simulink model "43_BusNetworkElectricityTransmissionModel"  (R2023b)
settings: Solver=VariableStepAuto  StartTime=0.0  StopTime=0.8  RelTol=1e-3
model workspace (MAT data in the model file):
  BESS_Fp_KDroop = 0.025
  BESS_KSI = 817
  BESS_PWM_fs = 560
  BESS_P_Ki = 0.5
  BESS_P_Kp = 0.0636
  BESS_Pnom = 3000000
  BESS_Q_Ki = 1
  BESS_Q_Kp = 0.0257
  BESS_Vd_Ki = 850
  BESS_Vd_Kp = 0.216
  BESS_Vnom = 1000
  BESS_Vq_KDroop = 0.025
  BESS_Vq_Ki = 850
  BESS_Vq_Kp = 0.216
  Compensation_Ki = 30
  Compensation_Kp = 3
  DC_Ki = 400
  DC_Kp = 8
  F = 0.01
  Flux_min = 0.5
  Grid_Freq_PWM = 2700
  Grid_Ireg_Ki = 5
  Grid_Ireg_Kp = 0.83
  Grid_Ireg_lim = 1.1
  Grid_Modindex_Upper = 1.1
  Grid_conv_Imax = 0.8
  H = 0.685
  Idref_max = 0.9
  Iqref_Tc = 0.3
  Ki_Var = 0.05
  Ki_Vreg = 20
  Ksh = 1.1
  L_pu = 0.3
  Llr = 0.16
  Lls = 0.18
  Lm = 2.9
  LowLoad_P = 130
  Nb_wt = 6
  P_mech = 1080000
  PeakShav_P = 200
  Pitch_Ki = 0
  Pitch_Kp = 150
  Pitch_Max = 27
  Pitch_Tc = 0.01
  Pitch_rate = 10
  Q_Filt = 50
  R_pu = 0.003
  Rotor_Freq_PWM = 1620
  Rotor_Ireg_Ki = 8
  Rotor_Ireg_Kp = 0.6
  Rotor_Ireg_lim = 0.1
  Rotor_Modindex_Upper = 2
  Rr = 0.016
  Rs = 0.023
  SOCBESS : Simulink.Parameter (value not decoded)
  T_set = 0.0001
  Tp = 5e-05
  Ts = 5e-06
  Var_C_Filt = 720000
  Var_reg_max = 1.1
  Var_reg_min = 0.9
  WT_Coeff = [0.645 116 0.4 5 21 0.00912 0.08 0.035]
  WT_H = 4.32
  WT_IGBTRon = 5.931
  WT_Param = [91.204 10143]
  Wind_Freq_Filt = 10000
  Wind_Freq_nom = 60
  Wind_P_nom = 1200000
  Wind_Rotor_V_nom = 1950
  Wind_V_nom = 500
  Zeta_Filt = 0.707106781187
  init = [-0.2 0 0 0 0 0 0 0]
  p = 3
  torque0 = 0.83
  v_Ki = 0.1
  v_Kp = 3.6
  v_Max = 1.2
  v_Min = 0.7
  v_T = 5
  vreg_max = 1
  wind_VDC_nom = 1150
  wt0 = 1.2
undefined symbols (not defined in the file): D1, D11, Delta, DiscIntNeverNeededParam, Iabc, Ion, Lithium, P, Q, Vabc
libraries: powerlib_extras x156, spsSeriesRLCBranchLib x66, spsLoadFlowBusLib x43, spsThreePhaseSeriesRLCLoadLib x33, spsThreePhaseTransformerTwoWindingsLib x32, spsThreePhaseVIMeasurementLib x30, simulink_extras x30, spsDistributedParametersLineLib x22, spsGenericPowerSystemStabilizerLib x20, spsSynchronousMachinepuStandardLib x10, spsExcitationSystemLib x10, spsHydraulicTurbineandGovernorLib x10
(part 7 of 19)

== system 43_BusNetworkElectricityTransmissionModel/South Network/Regulators 2 ==
  m : Inport
  Bus Selector : BusSelector  OutputSignals="dq0 components.Stator voltage  vq (pu),dq0 components.Stator voltage  vd (pu),Mechanical.Rotor speed  wm  (pu),Output active power   Peo (pu)"
  Constant : Constant  Value=0.8
  Constant1 : Constant
  Math Function : Math  Operator=hypot
  Turbine and Excitation Regulators : Subsystem
  Pm : Outport
  Vf : Outport  Port=2
  tag scope: Vm2=global, w2=global
  wires:
  Constant1/1 -> Turbine and Excitation Regulators/4(Vref)
  Turbine and Excitation Regulators/1(Pm) -> Pm/1
  m/1 -> Bus Selector/1
  Turbine and Excitation Regulators/2(Vf) -> Vf/1
  Bus Selector/1 -> Math Function/1  "<Stator voltage  vq (pu)>"
  Math Function/1 -> [Vm2], Turbine and Excitation Regulators/5(Vm)
  Bus Selector/2 -> Math Function/2  "<Stator voltage  vd (pu)>"
  Constant/1 -> Turbine and Excitation Regulators/1(pref)
  Bus Selector/3 -> [w2], Turbine and Excitation Regulators/2(w)  "<Rotor speed  wm  (pu)>"
  Bus Selector/4 -> Turbine and Excitation Regulators/3(Pe 0)  "<Output active power   Peo (pu)>"

== system 43_BusNetworkElectricityTransmissionModel/South Network/Regulators 3 ==
  m : Inport
  Bus Selector : BusSelector  OutputSignals="dq0 components.Stator voltage  vq (pu),dq0 components.Stator voltage  vd (pu),Mechanical.Rotor speed  wm  (pu),Output active power   Peo (pu)"
  Constant : Constant  Value=0.874
  Constant1 : Constant
  Math Function : Math  Operator=hypot
  Turbine and Excitation Regulators : Subsystem
  Pm : Outport
  Vf : Outport  Port=2
  tag scope: Vm3=global, w3=global
  wires:
  Bus Selector/4 -> Turbine and Excitation Regulators/3(Pe 0)  "<Output active power   Peo (pu)>"
  Constant1/1 -> Turbine and Excitation Regulators/4(Vref)
  Bus Selector/3 -> [w3], Turbine and Excitation Regulators/2(w)  "<Rotor speed  wm  (pu)>"
  Turbine and Excitation Regulators/1(Pm) -> Pm/1
  m/1 -> Bus Selector/1
  Turbine and Excitation Regulators/2(Vf) -> Vf/1
  Bus Selector/1 -> Math Function/1  "<Stator voltage  vq (pu)>"
  Math Function/1 -> [Vm3], Turbine and Excitation Regulators/5(Vm)
  Bus Selector/2 -> Math Function/2  "<Stator voltage  vd (pu)>"
  Constant/1 -> Turbine and Excitation Regulators/1(pref)

== system 43_BusNetworkElectricityTransmissionModel/South Network/Regulators 4 ==
  m : Inport
  Bus Selector : BusSelector  OutputSignals="dq0 components.Stator voltage  vq (pu),dq0 components.Stator voltage  vd (pu),Mechanical.Rotor speed  wm  (pu),Output active power   Peo (pu)"
  Constant : Constant  Value=0.842
  Constant1 : Constant
  Math Function : Math  Operator=hypot
  Turbine and Excitation Regulators : Subsystem
  Pm : Outport
  Vf : Outport  Port=2
  tag scope: Vm4=global, w4=global
  wires:
  Bus Selector/4 -> Turbine and Excitation Regulators/3(Pe 0)  "<Output active power   Peo (pu)>"
  Constant1/1 -> Turbine and Excitation Regulators/4(Vref)
  Bus Selector/3 -> [w4], Turbine and Excitation Regulators/2(w)  "<Rotor speed  wm  (pu)>"
  Turbine and Excitation Regulators/1(Pm) -> Pm/1
  m/1 -> Bus Selector/1
  Turbine and Excitation Regulators/2(Vf) -> Vf/1
  Bus Selector/1 -> Math Function/1  "<Stator voltage  vq (pu)>"
  Math Function/1 -> [Vm4], Turbine and Excitation Regulators/5(Vm)
  Bus Selector/2 -> Math Function/2  "<Stator voltage  vd (pu)>"
  Constant/1 -> Turbine and Excitation Regulators/1(pref)

== system 43_BusNetworkElectricityTransmissionModel/South Network/Regulators 5 ==
  m : Inport
  Bus Selector : BusSelector  OutputSignals="dq0 components.Stator voltage  vq (pu),dq0 components.Stator voltage  vd (pu),Mechanical.Rotor speed  wm  (pu),Output active power   Peo (pu)"
  Constant : Constant  Value=0.881
  Constant1 : Constant
  Math Function : Math  Operator=hypot
  Turbine and Excitation Regulators : Subsystem
  Pm : Outport
  Vf : Outport  Port=2
  tag scope: Vm5=global, w5=global
  wires:
  Constant1/1 -> Turbine and Excitation Regulators/4(Vref)
  Turbine and Excitation Regulators/1(Pm) -> Pm/1
  m/1 -> Bus Selector/1
  Turbine and Excitation Regulators/2(Vf) -> Vf/1
  Math Function/1 -> [Vm5], Turbine and Excitation Regulators/5(Vm)
  Constant/1 -> Turbine and Excitation Regulators/1(pref)
  Bus Selector/1 -> Math Function/1  "<Stator voltage  vq (pu)>"
  Bus Selector/2 -> Math Function/2  "<Stator voltage  vd (pu)>"
  Bus Selector/4 -> Turbine and Excitation Regulators/3(Pe 0)  "<Output active power   Peo (pu)>"
  Bus Selector/3 -> Turbine and Excitation Regulators/2(w), [w5]  "<Rotor speed  wm  (pu)>"

== system 43_BusNetworkElectricityTransmissionModel/South Network/Regulators 6 ==
  m : Inport
  Bus Selector : BusSelector  OutputSignals="dq0 components.Stator voltage  vq (pu),dq0 components.Stator voltage  vd (pu),Mechanical.Rotor speed  wm  (pu),Output active power   Peo (pu)"
  Constant : Constant  Value=0.847
  Constant1 : Constant
  Math Function : Math  Operator=hypot
  Turbine and Excitation Regulators : Subsystem
  Pm : Outport
  Vf : Outport  Port=2
  tag scope: Vm6=global, w6=global
  wires:
  Constant1/1 -> Turbine and Excitation Regulators/4(Vref)
  Turbine and Excitation Regulators/1(Pm) -> Pm/1
  m/1 -> Bus Selector/1
  Turbine and Excitation Regulators/2(Vf) -> Vf/1
  Math Function/1 -> [Vm6], Turbine and Excitation Regulators/5(Vm)
  Constant/1 -> Turbine and Excitation Regulators/1(pref)
  Bus Selector/1 -> Math Function/1  "<Stator voltage  vq (pu)>"
  Bus Selector/2 -> Math Function/2  "<Stator voltage  vd (pu)>"
  Bus Selector/4 -> Turbine and Excitation Regulators/3(Pe 0)  "<Output active power   Peo (pu)>"
  Bus Selector/3 -> Turbine and Excitation Regulators/2(w), [w6]  "<Rotor speed  wm  (pu)>"

== system 43_BusNetworkElectricityTransmissionModel/ 41.4 MW Wind Generation/41.4 MW Wind Farm/10.35 MW Wind Turbine 1 ==
  " base " : Gain  Gain=-P_mech/Wind_P_nom  SaturateOnIntegerOverflow=on  OutDataTypeStr=Inherit: Same as input  ParamDataTypeStr=Inherit: Same as input
  Asynchronous Machine pu Units : spsAsynchronousMachinepuUnitsLib/Asynchronous Machine pu Units  RotorType=Wound  PresetModel=No  MechanicalLoad=Torque Tm  ShowDetailedParameters=on  ReferenceFrame=Rotor  Units=pu  MeasurementBus=off  NominalParameters=[1.15e7 500 60]  VoltageRatio=1  Stator=[0.023 0.18]  Rotor=[0.016 0.16]  Cage1=[0.01909 0.0397]  Cage2=[0.01909 0.0397]  Lm=2.9  Mechanical=[0.685,0.01,3]  PolePairs=2  InitialConditions="[ -0.2,0   0,0,0   0,0,0 ]"  SimulateSaturation=off  Saturation="[0.212,0.4201,0.8125,1.0979,1.4799,2.2457,3.2586,4.5763,6.4763 ;   0.5,0.7,0.9,1,1.1,1.2 ,1.3,1.4,1.5]"  LoadFlowParameters=0  TsPowergui=0  TsBlock=-1  IterativeModel=Trapezoidal non iterative  IterativeDiscreteModel=Trapezoidal non iterative  Pmec=1.08e6
      settings: LibrarySourceBlock=|
      | sps_lib/Electrical Machines/Asynchronous Machine
      | pu Units
  Bus Selector : BusSelector  OutputSignals=Stator measurements.Stator current is_a (pu),Stator measurements.Stator current is_b (pu),Stator measurements.Stator current is_c (pu),Rotor measurements.Rotor current ir_a (pu),Rotor measurements.Rotor current ir_b (pu),Rotor measurements.Rotor current ir_c (pu),Mechanical.Electromagnetic torque Te (pu),Mechanical.Rotor speed (wm),Mechanical.Rotor angle thetam (rad)
  Mux : Mux  Inputs=3
  Mux1 : Mux  Inputs=3
  Series RLC Branch4 : spsSeriesRLCBranchLib/Series RLC Branch  LConnTagsString=__new0  RConnTagsString=__new0  BranchType=C  Resistance=1  Inductance=1e-3  SetiL0=off  InitialCurrent=0  Capacitance=4e-3  Setx0=on  InitialVoltage=1175  Measurements=None
  Three-Phase Series RLC Branch : spsThreePhaseSeriesRLCBranchLib/Three-Phase Series RLC Branch  LConnTagsString=A|B|C  RConnTagsString=A|B|C  BranchType=RL  Resistance=(Wind_V_nom^2/Wind_P_nom)*R_pu  Inductance=(Wind_V_nom^2/Wind_P_nom/(2*pi*Wind_Freq_nom))*L_pu  Capacitance=1e-6  Measurements=None
  Three-Phase Transformer (Two Windings) : spsThreePhaseTransformerTwoWindingsLib/Three-Phase Transformer (Two Windings)  Winding1Connection=Y  Winding2Connection=Y  CoreType=Three single-phase transformers  SetSaturation=off  Hysteresis=off  DataFile='hysteresis'  SetInitialFlux=off  Measurements=None  UNITS=pu  NominalPower=[1.15e7, 60 ]  Winding1="[ 500, 0,0  ]"  Winding2=[ 1950 , 0 , 0 ]  Rm=500  Lm=inf  L0=0.5  Saturation=[ 0,0 ; 0.0024,1.2 ; 1.0,1.52 ]  InitialFluxes=[ 0.8 , -0.8 , 0.7 ]  BreakLoop=off  DiscreteSolver=Trapezoidal iterative  DataType=off  TransfoNumber=1
  Three-Phase V-I Measurement5 : spsThreePhaseVIMeasurementLib/Three-Phase V-I Measurement  VoltageMeasurement=phase-to-ground  SetLabelV=on  LabelV=Rotor_Vabc_WT1  Vpu=on  VpuLL=off  CurrentMeasurement=no  SetLabelI=on  LabelI=Iabc_WT1  Ipu=on  Pbase=2*1.8/0.9  Vbase=Wind_Rotor_V_nom  OutputType=Complex  PhasorSimulation=off  PSBequivalent=0
  Three-Phase V-I Measurement6 : spsThreePhaseVIMeasurementLib/Three-Phase V-I Measurement  VoltageMeasurement=phase-to-ground  SetLabelV=on  LabelV=Grid_conv_Vabc_WT1  Vpu=on  VpuLL=off  CurrentMeasurement=yes  SetLabelI=on  LabelI=Grid_conv_Iabc_WT1  Ipu=on  Pbase=1.15e7  Vbase=Wind_V_nom  OutputType=Complex  PhasorSimulation=off  PSBequivalent=0
  Universal Bridge : spsUniversalBridgeLib/Universal Bridge  Arms=3  SnubberResistance=1e3  SnubberCapacitance=inf  Device=IGBT / Diodes  Ron=1e-4/WT_IGBTRon  Lon=0  ForwardVoltages="[  0  0  ]"  ForwardVoltage=0  GTOparameters=[ 10e-6 , 20e-6 ]  IGBTparameters=[ 1e-6 , 2e-6 ]  Measurements=None  Measurements_2=None  converterType=Rectifier
  Universal Bridge1 : spsUniversalBridgeLib/Universal Bridge  Arms=3  SnubberResistance=1e3  SnubberCapacitance=inf  Device=IGBT / Diodes  Ron=1e-4/WT_IGBTRon  Lon=0  ForwardVoltages="[  0  0  ]"  ForwardVoltage=0  GTOparameters=[ 10e-6 , 20e-6 ]  IGBTparameters=[ 1e-6 , 2e-6 ]  Measurements=None  Measurements_2=None  converterType=Rectifier
  Wind Turbine & Generator 1 : Subsystem
  A : PMIOPort  Side=Left
  B : PMIOPort  Port=2  Side=Left
  C : PMIOPort  Port=3  Side=Left
  tag scope: Rotor_Angle_WT1=global, Rotor_Iabc_WT1=global, Rotor_Tem_WT1=global, Rotor_wm_WT1=global, Stator_Iabc_WT1=global, Tshaft_WT1=global, m_WT1=global
  wires:
  [Tshaft_WT1] -> Asynchronous Machine pu Units/1
  Wind Turbine & Generator 1/1(T_shaft (pu)) -> " base "/1
  " base "/1 -> [Tshaft_WT1]
  Asynchronous Machine pu Units/1 -> [m_WT1]
  [Grid_conv_pulses_WT1] -> Universal Bridge1/1
  [Rotor_conv_pulses_WT1] -> Universal Bridge/1
  [Rotor_wm_WT1] -> Wind Turbine & Generator 1/1(Generator speed (pu))
  [m_WT1] -> Bus Selector/1
  Bus Selector/1 -> Mux1/1  "<Stator current is_a (pu)>"
  Bus Selector/2 -> Mux1/2  "<Stator current is_b (pu)>"
  Bus Selector/3 -> Mux1/3  "<Stator current is_c (pu)>"
  Bus Selector/4 -> Mux/1  "<Rotor current ir_a (pu)>"
  Bus Selector/5 -> Mux/2  "<Rotor current ir_b (pu)>"
  Bus Selector/6 -> Mux/3  "<Rotor current ir_c (pu)>"
  Bus Selector/7 -> [Rotor_Tem_WT1]  "<Electromagnetic torque Te (pu)>"
  Bus Selector/8 -> [Rotor_wm_WT1]  "<Rotor speed (wm)>"
  Bus Selector/9 -> [Rotor_Angle_WT1]  "<Rotor angle thetam (rad)>"
  Mux/1 -> [Rotor_Iabc_WT1]
  Mux1/1 -> [Stator_Iabc_WT1]
  connections:
  Asynchronous Machine pu Units/LConn3 -- C/RConn1 -- Three-Phase Series RLC Branch/LConn3
  Three-Phase Series RLC Branch/LConn1 -- A/RConn1 -- Asynchronous Machine pu Units/LConn1
  Three-Phase Transformer (Two Windings)/LConn1 -- Asynchronous Machine pu Units/RConn1
  Three-Phase Transformer (Two Windings)/RConn1 -- Three-Phase V-I Measurement5/LConn1
  Three-Phase Series RLC Branch/LConn2 -- B/RConn1 -- Asynchronous Machine pu Units/LConn2
  Universal Bridge1/LConn3 -- Three-Phase V-I Measurement6/RConn3
  Three-Phase Transformer (Two Windings)/LConn3 -- Asynchronous Machine pu Units/RConn3
  Three-Phase Transformer (Two Windings)/LConn2 -- Asynchronous Machine pu Units/RConn2
  Universal Bridge1/LConn2 -- Three-Phase V-I Measurement6/RConn2
  Universal Bridge/RConn1 -- Series RLC Branch4/LConn1 -- Universal Bridge1/RConn1
  Universal Bridge1/RConn2 -- Series RLC Branch4/RConn1 -- Universal Bridge/RConn2
  Three-Phase Transformer (Two Windings)/RConn2 -- Three-Phase V-I Measurement5/LConn2
  Three-Phase V-I Measurement5/RConn3 -- Universal Bridge/LConn3
  Three-Phase V-I Measurement5/RConn1 -- Universal Bridge/LConn1
  Three-Phase Transformer (Two Windings)/RConn3 -- Three-Phase V-I Measurement5/LConn3
  Three-Phase V-I Measurement6/LConn1 -- Three-Phase Series RLC Branch/RConn1
  Three-Phase Series RLC Branch/RConn2 -- Three-Phase V-I Measurement6/LConn2
  Universal Bridge1/LConn1 -- Three-Phase V-I Measurement6/RConn1
  Three-Phase Series RLC Branch/RConn3 -- Three-Phase V-I Measurement6/LConn3
  Three-Phase V-I Measurement5/RConn2 -- Universal Bridge/LConn2

== system 43_BusNetworkElectricityTransmissionModel/ 41.4 MW Wind Generation/41.4 MW Wind Farm/10.35 MW Wind Turbine 2 ==
  " base " : Gain  Gain=-P_mech/Wind_P_nom  SaturateOnIntegerOverflow=on  OutDataTypeStr=Inherit: Same as input  ParamDataTypeStr=Inherit: Same as input
  Asynchronous Machine pu Units : spsAsynchronousMachinepuUnitsLib/Asynchronous Machine pu Units  RotorType=Wound  PresetModel=No  MechanicalLoad=Torque Tm  ShowDetailedParameters=on  ReferenceFrame=Rotor  Units=pu  MeasurementBus=off  NominalParameters=[1.15e7 500 60]  VoltageRatio=1  Stator=[0.023 0.18]  Rotor=[0.016 0.16]  Cage1=[0.01909 0.0397]  Cage2=[0.01909 0.0397]  Lm=2.9  Mechanical=[0.685,0.01,3]  PolePairs=2  InitialConditions="[ -0.2,0   0,0,0   0,0,0 ]"  SimulateSaturation=off  Saturation="[0.212,0.4201,0.8125,1.0979,1.4799,2.2457,3.2586,4.5763,6.4763 ;   0.5,0.7,0.9,1,1.1,1.2 ,1.3,1.4,1.5]"  LoadFlowParameters=0  TsPowergui=0  TsBlock=-1  IterativeModel=Trapezoidal non iterative  IterativeDiscreteModel=Trapezoidal non iterative  Pmec=1.08e6
      settings: LibrarySourceBlock=|
      | sps_lib/Electrical Machines/Asynchronous Machine
      | pu Units
  Bus Selector : BusSelector  OutputSignals=Stator measurements.Stator current is_a (pu),Stator measurements.Stator current is_b (pu),Stator measurements.Stator current is_c (pu),Rotor measurements.Rotor current ir_a (pu),Rotor measurements.Rotor current ir_b (pu),Rotor measurements.Rotor current ir_c (pu),Mechanical.Electromagnetic torque Te (pu),Mechanical.Rotor speed (wm),Mechanical.Rotor angle thetam (rad)
  Mux : Mux  Inputs=3
  Mux1 : Mux  Inputs=3
  Series RLC Branch4 : spsSeriesRLCBranchLib/Series RLC Branch  LConnTagsString=__new0  RConnTagsString=__new0  BranchType=C  Resistance=1  Inductance=1e-3  SetiL0=off  InitialCurrent=0  Capacitance=4e-3  Setx0=on  InitialVoltage=1175  Measurements=None
  Three-Phase Series RLC Branch : spsThreePhaseSeriesRLCBranchLib/Three-Phase Series RLC Branch  LConnTagsString=A|B|C  RConnTagsString=A|B|C  BranchType=RL  Resistance=(Wind_V_nom^2/Wind_P_nom)*R_pu  Inductance=(Wind_V_nom^2/Wind_P_nom/(2*pi*Wind_Freq_nom))*L_pu  Capacitance=1e-6  Measurements=None
  Three-Phase Transformer (Two Windings) : spsThreePhaseTransformerTwoWindingsLib/Three-Phase Transformer (Two Windings)  Winding1Connection=Y  Winding2Connection=Y  CoreType=Three single-phase transformers  SetSaturation=off  Hysteresis=off  DataFile='hysteresis'  SetInitialFlux=off  Measurements=None  UNITS=pu  NominalPower=[1.15e7, 60 ]  Winding1="[ 500, 0,0  ]"  Winding2=[ 1950 , 0 , 0 ]  Rm=500  Lm=inf  L0=0.5  Saturation=[ 0,0 ; 0.0024,1.2 ; 1.0,1.52 ]  InitialFluxes=[ 0.8 , -0.8 , 0.7 ]  BreakLoop=off  DiscreteSolver=Trapezoidal iterative  DataType=off  TransfoNumber=1
  Three-Phase V-I Measurement5 : spsThreePhaseVIMeasurementLib/Three-Phase V-I Measurement  VoltageMeasurement=phase-to-ground  SetLabelV=on  LabelV=Rotor_Vabc_WT2  Vpu=on  VpuLL=off  CurrentMeasurement=no  SetLabelI=on  LabelI=Iabc_WT1  Ipu=on  Pbase=2*1.8/0.9  Vbase=Wind_Rotor_V_nom  OutputType=Complex  PhasorSimulation=off  PSBequivalent=0
  Three-Phase V-I Measurement6 : spsThreePhaseVIMeasurementLib/Three-Phase V-I Measurement  VoltageMeasurement=phase-to-ground  SetLabelV=on  LabelV=Grid_conv_Vabc_WT2  Vpu=on  VpuLL=off  CurrentMeasurement=yes  SetLabelI=on  LabelI=Grid_conv_Iabc_WT2  Ipu=on  Pbase=1.15e7  Vbase=Wind_V_nom  OutputType=Complex  PhasorSimulation=off  PSBequivalent=0
  Universal Bridge : spsUniversalBridgeLib/Universal Bridge  Arms=3  SnubberResistance=1e3  SnubberCapacitance=inf  Device=IGBT / Diodes  Ron=1e-4/WT_IGBTRon  Lon=0  ForwardVoltages="[  0  0  ]"  ForwardVoltage=0  GTOparameters=[ 10e-6 , 20e-6 ]  IGBTparameters=[ 1e-6 , 2e-6 ]  Measurements=None  Measurements_2=None  converterType=Rectifier
  Universal Bridge1 : spsUniversalBridgeLib/Universal Bridge  Arms=3  SnubberResistance=1e3  SnubberCapacitance=inf  Device=IGBT / Diodes  Ron=1e-4/WT_IGBTRon  Lon=0  ForwardVoltages="[  0  0  ]"  ForwardVoltage=0  GTOparameters=[ 10e-6 , 20e-6 ]  IGBTparameters=[ 1e-6 , 2e-6 ]  Measurements=None  Measurements_2=None  converterType=Rectifier
  Wind Turbine & Generator 1 : Subsystem
  A : PMIOPort  Side=Left
  B : PMIOPort  Port=2  Side=Left
  C : PMIOPort  Port=3  Side=Left
  tag scope: Rotor_Angle_WT2=global, Rotor_Iabc_WT2=global, Rotor_Tem_WT2=global, Rotor_wm_WT2=global, Stator_Iabc_WT2=global, Tshaft_WT2=global, m_WT2=global
  wires:
  [Tshaft_WT2] -> Asynchronous Machine pu Units/1
  Wind Turbine & Generator 1/1(T_shaft (pu)) -> " base "/1
  " base "/1 -> [Tshaft_WT2]
  Asynchronous Machine pu Units/1 -> [m_WT2]
  [Grid_conv_pulses_WT2] -> Universal Bridge1/1
  [Rotor_conv_pulses_WT2] -> Universal Bridge/1
  [Rotor_wm_WT2] -> Wind Turbine & Generator 1/1(Generator speed (pu))
  [m_WT2] -> Bus Selector/1
  Bus Selector/1 -> Mux1/1  "<Stator current is_a (pu)>"
  Bus Selector/2 -> Mux1/2  "<Stator current is_b (pu)>"
  Bus Selector/3 -> Mux1/3  "<Stator current is_c (pu)>"
  Bus Selector/4 -> Mux/1  "<Rotor current ir_a (pu)>"
  Bus Selector/5 -> Mux/2  "<Rotor current ir_b (pu)>"
  Bus Selector/6 -> Mux/3  "<Rotor current ir_c (pu)>"
  Bus Selector/7 -> [Rotor_Tem_WT2]  "<Electromagnetic torque Te (pu)>"
  Bus Selector/8 -> [Rotor_wm_WT2]  "<Rotor speed (wm)>"
  Bus Selector/9 -> [Rotor_Angle_WT2]  "<Rotor angle thetam (rad)>"
  Mux/1 -> [Rotor_Iabc_WT2]
  Mux1/1 -> [Stator_Iabc_WT2]
  connections:
  Asynchronous Machine pu Units/LConn3 -- C/RConn1 -- Three-Phase Series RLC Branch/LConn3
  Three-Phase Series RLC Branch/LConn1 -- A/RConn1 -- Asynchronous Machine pu Units/LConn1
  Three-Phase Transformer (Two Windings)/LConn1 -- Asynchronous Machine pu Units/RConn1
  Three-Phase Transformer (Two Windings)/RConn1 -- Three-Phase V-I Measurement5/LConn1
  Three-Phase Series RLC Branch/LConn2 -- B/RConn1 -- Asynchronous Machine pu Units/LConn2
  Universal Bridge1/LConn3 -- Three-Phase V-I Measurement6/RConn3
  Three-Phase Transformer (Two Windings)/LConn3 -- Asynchronous Machine pu Units/RConn3
  Three-Phase Transformer (Two Windings)/LConn2 -- Asynchronous Machine pu Units/RConn2
  Universal Bridge1/LConn2 -- Three-Phase V-I Measurement6/RConn2
  Universal Bridge/RConn1 -- Series RLC Branch4/LConn1 -- Universal Bridge1/RConn1
  Universal Bridge1/RConn2 -- Series RLC Branch4/RConn1 -- Universal Bridge/RConn2
  Three-Phase Transformer (Two Windings)/RConn2 -- Three-Phase V-I Measurement5/LConn2
  Three-Phase V-I Measurement5/RConn3 -- Universal Bridge/LConn3
  Three-Phase V-I Measurement5/RConn1 -- Universal Bridge/LConn1
  Three-Phase Transformer (Two Windings)/RConn3 -- Three-Phase V-I Measurement5/LConn3
  Three-Phase V-I Measurement6/LConn1 -- Three-Phase Series RLC Branch/RConn1
  Three-Phase Series RLC Branch/RConn2 -- Three-Phase V-I Measurement6/LConn2
  Universal Bridge1/LConn1 -- Three-Phase V-I Measurement6/RConn1
  Three-Phase Series RLC Branch/RConn3 -- Three-Phase V-I Measurement6/LConn3
  Three-Phase V-I Measurement5/RConn2 -- Universal Bridge/LConn2

== system 43_BusNetworkElectricityTransmissionModel/ 41.4 MW Wind Generation/41.4 MW Wind Farm/10.35 MW Wind Turbine 3 ==
  " base " : Gain  Gain=-P_mech/Wind_P_nom  SaturateOnIntegerOverflow=on  OutDataTypeStr=Inherit: Same as input  ParamDataTypeStr=Inherit: Same as input
  Asynchronous Machine pu Units : spsAsynchronousMachinepuUnitsLib/Asynchronous Machine pu Units  RotorType=Wound  PresetModel=No  MechanicalLoad=Torque Tm  ShowDetailedParameters=on  ReferenceFrame=Rotor  Units=pu  MeasurementBus=off  NominalParameters=[1.15e7 500 60]  VoltageRatio=1  Stator=[0.023 0.18]  Rotor=[0.016 0.16]  Cage1=[0.01909 0.0397]  Cage2=[0.01909 0.0397]  Lm=2.9  Mechanical=[0.685,0.01,3]  PolePairs=2  InitialConditions="[ -0.2,0   0,0,0   0,0,0 ]"  SimulateSaturation=off  Saturation="[0.212,0.4201,0.8125,1.0979,1.4799,2.2457,3.2586,4.5763,6.4763 ;   0.5,0.7,0.9,1,1.1,1.2 ,1.3,1.4,1.5]"  LoadFlowParameters=0  TsPowergui=0  TsBlock=-1  IterativeModel=Trapezoidal non iterative  IterativeDiscreteModel=Trapezoidal non iterative  Pmec=1.08e6
      settings: LibrarySourceBlock=|
      | sps_lib/Electrical Machines/Asynchronous Machine
      | pu Units
  Bus Selector : BusSelector  OutputSignals=Stator measurements.Stator current is_a (pu),Stator measurements.Stator current is_b (pu),Stator measurements.Stator current is_c (pu),Rotor measurements.Rotor current ir_a (pu),Rotor measurements.Rotor current ir_b (pu),Rotor measurements.Rotor current ir_c (pu),Mechanical.Electromagnetic torque Te (pu),Mechanical.Rotor speed (wm),Mechanical.Rotor angle thetam (rad)
  Mux : Mux  Inputs=3
  Mux1 : Mux  Inputs=3
  Series RLC Branch4 : spsSeriesRLCBranchLib/Series RLC Branch  LConnTagsString=__new0  RConnTagsString=__new0  BranchType=C  Resistance=1  Inductance=1e-3  SetiL0=off  InitialCurrent=0  Capacitance=4e-3  Setx0=on  InitialVoltage=1175  Measurements=None
  Three-Phase Series RLC Branch : spsThreePhaseSeriesRLCBranchLib/Three-Phase Series RLC Branch  LConnTagsString=A|B|C  RConnTagsString=A|B|C  BranchType=RL  Resistance=(Wind_V_nom^2/Wind_P_nom)*R_pu  Inductance=(Wind_V_nom^2/Wind_P_nom/(2*pi*Wind_Freq_nom))*L_pu  Capacitance=1e-6  Measurements=None
  Three-Phase Transformer (Two Windings) : spsThreePhaseTransformerTwoWindingsLib/Three-Phase Transformer (Two Windings)  Winding1Connection=Y  Winding2Connection=Y  CoreType=Three single-phase transformers  SetSaturation=off  Hysteresis=off  DataFile='hysteresis'  SetInitialFlux=off  Measurements=None  UNITS=pu  NominalPower=[1.15e7, 60 ]  Winding1="[ 500, 0,0  ]"  Winding2=[ 1950 , 0 , 0 ]  Rm=500  Lm=inf  L0=0.5  Saturation=[ 0,0 ; 0.0024,1.2 ; 1.0,1.52 ]  InitialFluxes=[ 0.8 , -0.8 , 0.7 ]  BreakLoop=off  DiscreteSolver=Trapezoidal iterative  DataType=off  TransfoNumber=1
  Three-Phase V-I Measurement5 : spsThreePhaseVIMeasurementLib/Three-Phase V-I Measurement  VoltageMeasurement=phase-to-ground  SetLabelV=on  LabelV=Rotor_Vabc_WT3  Vpu=on  VpuLL=off  CurrentMeasurement=no  SetLabelI=on  LabelI=Iabc_WT1  Ipu=on  Pbase=2*1.8/0.9  Vbase=Wind_Rotor_V_nom  OutputType=Complex  PhasorSimulation=off  PSBequivalent=0
  Three-Phase V-I Measurement6 : spsThreePhaseVIMeasurementLib/Three-Phase V-I Measurement  VoltageMeasurement=phase-to-ground  SetLabelV=on  LabelV=Grid_conv_Vabc_WT3  Vpu=on  VpuLL=off  CurrentMeasurement=yes  SetLabelI=on  LabelI=Grid_conv_Iabc_WT3  Ipu=on  Pbase=1.15e7  Vbase=Wind_V_nom  OutputType=Complex  PhasorSimulation=off  PSBequivalent=0
  Universal Bridge : spsUniversalBridgeLib/Universal Bridge  Arms=3  SnubberResistance=1e3  SnubberCapacitance=inf  Device=IGBT / Diodes  Ron=1e-4/WT_IGBTRon  Lon=0  ForwardVoltages="[  0  0  ]"  ForwardVoltage=0  GTOparameters=[ 10e-6 , 20e-6 ]  IGBTparameters=[ 1e-6 , 2e-6 ]  Measurements=None  Measurements_2=None  converterType=Rectifier
  Universal Bridge1 : spsUniversalBridgeLib/Universal Bridge  Arms=3  SnubberResistance=1e3  SnubberCapacitance=inf  Device=IGBT / Diodes  Ron=1e-4/WT_IGBTRon  Lon=0  ForwardVoltages="[  0  0  ]"  ForwardVoltage=0  GTOparameters=[ 10e-6 , 20e-6 ]  IGBTparameters=[ 1e-6 , 2e-6 ]  Measurements=None  Measurements_2=None  converterType=Rectifier
  Wind Turbine & Generator 1 : Subsystem
  A : PMIOPort  Side=Left
  B : PMIOPort  Port=2  Side=Left
  C : PMIOPort  Port=3  Side=Left
  tag scope: Rotor_Angle_WT3=global, Rotor_Iabc_WT3=global, Rotor_Tem_WT3=global, Rotor_wm_WT3=global, Stator_Iabc_WT3=global, Tshaft_WT3=global, m_WT3=global
  wires:
  [Tshaft_WT3] -> Asynchronous Machine pu Units/1
  Wind Turbine & Generator 1/1(T_shaft (pu)) -> " base "/1
  " base "/1 -> [Tshaft_WT3]
  Asynchronous Machine pu Units/1 -> [m_WT3]
  [Grid_conv_pulses_WT3] -> Universal Bridge1/1
  [Rotor_conv_pulses_WT3] -> Universal Bridge/1
  [Rotor_wm_WT3] -> Wind Turbine & Generator 1/1(Generator speed (pu))
  [m_WT3] -> Bus Selector/1
  Bus Selector/1 -> Mux1/1  "<Stator current is_a (pu)>"
  Bus Selector/2 -> Mux1/2  "<Stator current is_b (pu)>"
  Bus Selector/3 -> Mux1/3  "<Stator current is_c (pu)>"
  Bus Selector/4 -> Mux/1  "<Rotor current ir_a (pu)>"
  Bus Selector/5 -> Mux/2  "<Rotor current ir_b (pu)>"
  Bus Selector/6 -> Mux/3  "<Rotor current ir_c (pu)>"
  Bus Selector/7 -> [Rotor_Tem_WT3]  "<Electromagnetic torque Te (pu)>"
  Bus Selector/8 -> [Rotor_wm_WT3]  "<Rotor speed (wm)>"
  Bus Selector/9 -> [Rotor_Angle_WT3]  "<Rotor angle thetam (rad)>"
  Mux/1 -> [Rotor_Iabc_WT3]
  Mux1/1 -> [Stator_Iabc_WT3]
  connections:
  Asynchronous Machine pu Units/LConn3 -- C/RConn1 -- Three-Phase Series RLC Branch/LConn3
  Three-Phase Series RLC Branch/LConn1 -- A/RConn1 -- Asynchronous Machine pu Units/LConn1
  Three-Phase Transformer (Two Windings)/LConn1 -- Asynchronous Machine pu Units/RConn1
  Three-Phase Transformer (Two Windings)/RConn1 -- Three-Phase V-I Measurement5/LConn1
  Three-Phase Series RLC Branch/LConn2 -- B/RConn1 -- Asynchronous Machine pu Units/LConn2
  Universal Bridge1/LConn3 -- Three-Phase V-I Measurement6/RConn3
  Three-Phase Transformer (Two Windings)/LConn3 -- Asynchronous Machine pu Units/RConn3
  Three-Phase Transformer (Two Windings)/LConn2 -- Asynchronous Machine pu Units/RConn2
  Universal Bridge1/LConn2 -- Three-Phase V-I Measurement6/RConn2
  Universal Bridge/RConn1 -- Series RLC Branch4/LConn1 -- Universal Bridge1/RConn1
  Universal Bridge1/RConn2 -- Series RLC Branch4/RConn1 -- Universal Bridge/RConn2
  Three-Phase Transformer (Two Windings)/RConn2 -- Three-Phase V-I Measurement5/LConn2
  Three-Phase V-I Measurement5/RConn3 -- Universal Bridge/LConn3
  Three-Phase V-I Measurement5/RConn1 -- Universal Bridge/LConn1
  Three-Phase Transformer (Two Windings)/RConn3 -- Three-Phase V-I Measurement5/LConn3
  Three-Phase V-I Measurement6/LConn1 -- Three-Phase Series RLC Branch/RConn1
  Three-Phase Series RLC Branch/RConn2 -- Three-Phase V-I Measurement6/LConn2
  Universal Bridge1/LConn1 -- Three-Phase V-I Measurement6/RConn1
  Three-Phase Series RLC Branch/RConn3 -- Three-Phase V-I Measurement6/LConn3
  Three-Phase V-I Measurement5/RConn2 -- Universal Bridge/LConn2

== system 43_BusNetworkElectricityTransmissionModel/ 41.4 MW Wind Generation/41.4 MW Wind Farm/10.35 MW Wind Turbine 4 ==
  " base " : Gain  Gain=-P_mech/Wind_P_nom  SaturateOnIntegerOverflow=on  OutDataTypeStr=Inherit: Same as input  ParamDataTypeStr=Inherit: Same as input
  Asynchronous Machine pu Units : spsAsynchronousMachinepuUnitsLib/Asynchronous Machine pu Units  RotorType=Wound  PresetModel=No  MechanicalLoad=Torque Tm  ShowDetailedParameters=on  ReferenceFrame=Rotor  Units=pu  MeasurementBus=off  NominalParameters=[1.15e7 500 60]  VoltageRatio=1  Stator=[0.023 0.18]  Rotor=[0.016 0.16]  Cage1=[0.01909 0.0397]  Cage2=[0.01909 0.0397]  Lm=2.9  Mechanical=[0.685,0.01,3]  PolePairs=2  InitialConditions="[ -0.2,0   0,0,0   0,0,0 ]"  SimulateSaturation=off  Saturation="[0.212,0.4201,0.8125,1.0979,1.4799,2.2457,3.2586,4.5763,6.4763 ;   0.5,0.7,0.9,1,1.1,1.2 ,1.3,1.4,1.5]"  LoadFlowParameters=0  TsPowergui=0  TsBlock=-1  IterativeModel=Trapezoidal non iterative  IterativeDiscreteModel=Trapezoidal non iterative  Pmec=1.08e6
      settings: LibrarySourceBlock=|
      | sps_lib/Electrical Machines/Asynchronous Machine
      | pu Units
  Bus Selector : BusSelector  OutputSignals=Stator measurements.Stator current is_a (pu),Stator measurements.Stator current is_b (pu),Stator measurements.Stator current is_c (pu),Rotor measurements.Rotor current ir_a (pu),Rotor measurements.Rotor current ir_b (pu),Rotor measurements.Rotor current ir_c (pu),Mechanical.Electromagnetic torque Te (pu),Mechanical.Rotor speed (wm),Mechanical.Rotor angle thetam (rad)
  Mux : Mux  Inputs=3
  Mux1 : Mux  Inputs=3
  Series RLC Branch4 : spsSeriesRLCBranchLib/Series RLC Branch  LConnTagsString=__new0  RConnTagsString=__new0  BranchType=C  Resistance=1  Inductance=1e-3  SetiL0=off  InitialCurrent=0  Capacitance=4e-3  Setx0=on  InitialVoltage=1175  Measurements=None
  Three-Phase Series RLC Branch : spsThreePhaseSeriesRLCBranchLib/Three-Phase Series RLC Branch  LConnTagsString=A|B|C  RConnTagsString=A|B|C  BranchType=RL  Resistance=(Wind_V_nom^2/Wind_P_nom)*R_pu  Inductance=(Wind_V_nom^2/Wind_P_nom/(2*pi*Wind_Freq_nom))*L_pu  Capacitance=1e-6  Measurements=None
  Three-Phase Transformer (Two Windings) : spsThreePhaseTransformerTwoWindingsLib/Three-Phase Transformer (Two Windings)  Winding1Connection=Y  Winding2Connection=Y  CoreType=Three single-phase transformers  SetSaturation=off  Hysteresis=off  DataFile='hysteresis'  SetInitialFlux=off  Measurements=None  UNITS=pu  NominalPower=[1.15e7, 60 ]  Winding1="[ 500, 0,0  ]"  Winding2=[ 1950 , 0 , 0 ]  Rm=500  Lm=inf  L0=0.5  Saturation=[ 0,0 ; 0.0024,1.2 ; 1.0,1.52 ]  InitialFluxes=[ 0.8 , -0.8 , 0.7 ]  BreakLoop=off  DiscreteSolver=Trapezoidal iterative  DataType=off  TransfoNumber=1
  Three-Phase V-I Measurement5 : spsThreePhaseVIMeasurementLib/Three-Phase V-I Measurement  VoltageMeasurement=phase-to-ground  SetLabelV=on  LabelV=Rotor_Vabc_WT4  Vpu=on  VpuLL=off  CurrentMeasurement=no  SetLabelI=on  LabelI=Iabc_WT1  Ipu=on  Pbase=2*1.8/0.9  Vbase=Wind_Rotor_V_nom  OutputType=Complex  PhasorSimulation=off  PSBequivalent=0
  Three-Phase V-I Measurement6 : spsThreePhaseVIMeasurementLib/Three-Phase V-I Measurement  VoltageMeasurement=phase-to-ground  SetLabelV=on  LabelV=Grid_conv_Vabc_WT4  Vpu=on  VpuLL=off  CurrentMeasurement=yes  SetLabelI=on  LabelI=Grid_conv_Iabc_WT4  Ipu=on  Pbase=1.15e7  Vbase=Wind_V_nom  OutputType=Complex  PhasorSimulation=off  PSBequivalent=0
  Universal Bridge : spsUniversalBridgeLib/Universal Bridge  Arms=3  SnubberResistance=1e3  SnubberCapacitance=inf  Device=IGBT / Diodes  Ron=1e-4/WT_IGBTRon  Lon=0  ForwardVoltages="[  0  0  ]"  ForwardVoltage=0  GTOparameters=[ 10e-6 , 20e-6 ]  IGBTparameters=[ 1e-6 , 2e-6 ]  Measurements=None  Measurements_2=None  converterType=Rectifier
  Universal Bridge1 : spsUniversalBridgeLib/Universal Bridge  Arms=3  SnubberResistance=1e3  SnubberCapacitance=inf  Device=IGBT / Diodes  Ron=1e-4/WT_IGBTRon  Lon=0  ForwardVoltages="[  0  0  ]"  ForwardVoltage=0  GTOparameters=[ 10e-6 , 20e-6 ]  IGBTparameters=[ 1e-6 , 2e-6 ]  Measurements=None  Measurements_2=None  converterType=Rectifier
  Wind Turbine & Generator 1 : Subsystem
  A : PMIOPort  Side=Left
  B : PMIOPort  Port=2  Side=Left
  C : PMIOPort  Port=3  Side=Left
  tag scope: Rotor_Angle_WT4=global, Rotor_Iabc_WT4=global, Rotor_Tem_WT4=global, Rotor_wm_WT4=global, Stator_Iabc_WT4=global, Tshaft_WT4=global, m_WT4=global
  wires:
  [Tshaft_WT4] -> Asynchronous Machine pu Units/1
  Wind Turbine & Generator 1/1(T_shaft (pu)) -> " base "/1
  " base "/1 -> [Tshaft_WT4]
  Asynchronous Machine pu Units/1 -> [m_WT4]
  [Grid_conv_pulses_WT4] -> Universal Bridge1/1
  [Rotor_conv_pulses_WT4] -> Universal Bridge/1
  [Rotor_wm_WT4] -> Wind Turbine & Generator 1/1(Generator speed (pu))
  [m_WT4] -> Bus Selector/1
  Bus Selector/1 -> Mux1/1  "<Stator current is_a (pu)>"
  Bus Selector/2 -> Mux1/2  "<Stator current is_b (pu)>"
  Bus Selector/3 -> Mux1/3  "<Stator current is_c (pu)>"
  Bus Selector/4 -> Mux/1  "<Rotor current ir_a (pu)>"
  Bus Selector/5 -> Mux/2  "<Rotor current ir_b (pu)>"
  Bus Selector/6 -> Mux/3  "<Rotor current ir_c (pu)>"
  Bus Selector/7 -> [Rotor_Tem_WT4]  "<Electromagnetic torque Te (pu)>"
  Bus Selector/8 -> [Rotor_wm_WT4]  "<Rotor speed (wm)>"
  Bus Selector/9 -> [Rotor_Angle_WT4]  "<Rotor angle thetam (rad)>"
  Mux/1 -> [Rotor_Iabc_WT4]
  Mux1/1 -> [Stator_Iabc_WT4]
  connections:
  Asynchronous Machine pu Units/LConn3 -- C/RConn1 -- Three-Phase Series RLC Branch/LConn3
  Three-Phase Series RLC Branch/LConn1 -- A/RConn1 -- Asynchronous Machine pu Units/LConn1
  Three-Phase Transformer (Two Windings)/LConn1 -- Asynchronous Machine pu Units/RConn1
  Three-Phase Transformer (Two Windings)/RConn1 -- Three-Phase V-I Measurement5/LConn1
  Three-Phase Series RLC Branch/LConn2 -- B/RConn1 -- Asynchronous Machine pu Units/LConn2
  Universal Bridge1/LConn3 -- Three-Phase V-I Measurement6/RConn3
  Three-Phase Transformer (Two Windings)/LConn3 -- Asynchronous Machine pu Units/RConn3
  Three-Phase Transformer (Two Windings)/LConn2 -- Asynchronous Machine pu Units/RConn2
  Universal Bridge1/LConn2 -- Three-Phase V-I Measurement6/RConn2
  Universal Bridge/RConn1 -- Series RLC Branch4/LConn1 -- Universal Bridge1/RConn1
  Universal Bridge1/RConn2 -- Series RLC Branch4/RConn1 -- Universal Bridge/RConn2
  Three-Phase Transformer (Two Windings)/RConn2 -- Three-Phase V-I Measurement5/LConn2
  Three-Phase V-I Measurement5/RConn3 -- Universal Bridge/LConn3
  Three-Phase V-I Measurement5/RConn1 -- Universal Bridge/LConn1
  Three-Phase Transformer (Two Windings)/RConn3 -- Three-Phase V-I Measurement5/LConn3
  Three-Phase V-I Measurement6/LConn1 -- Three-Phase Series RLC Branch/RConn1
  Three-Phase Series RLC Branch/RConn2 -- Three-Phase V-I Measurement6/LConn2
  Universal Bridge1/LConn1 -- Three-Phase V-I Measurement6/RConn1
  Three-Phase Series RLC Branch/RConn3 -- Three-Phase V-I Measurement6/LConn3
  Three-Phase V-I Measurement5/RConn2 -- Universal Bridge/LConn2

== system 43_BusNetworkElectricityTransmissionModel/ 41.4 MW Wind Generation/41.4 MW Wind Farm/Control System ==
  Control System 1 : Subsystem
  Control System 2 : Subsystem
  Control System 3 : Subsystem
  Control System 4 : Subsystem
  tag scope: Grid_conv_pulses_WT1=global, Grid_conv_pulses_WT2=global, Grid_conv_pulses_WT3=global, Grid_conv_pulses_WT4=global, PQ_WT1=global, PQ_WT2=global, PQ_WT3=global, PQ_WT4=global, Pitch_WT1=global, Pitch_WT2=global, Pitch_WT3=global, Pitch_WT4=global, Rotor_conv_pulses_WT1=global, Rotor_conv_pulses_WT2=global, Rotor_conv_pulses_WT3=global, Rotor_conv_pulses_WT4=global
  wires:
  [Vabc_WT1] -> Control System 1/1(Vabc)
  Control System 4/1(Grid_conv_pulses) -> [Grid_conv_pulses_WT4]
  [Stator_Iabc_WT4] -> Control System 4/2(Stator_Iabc)
  [Grid_conv_Iabc_WT3] -> Control System 3/3(Grid_Iabc)
  [Q_ref_WT2] -> Control System 2/6(Qref1)
  [Rotor_wm_WT1] -> Control System 1/8(wr)
  Control System 1/3(Pitch) -> [Pitch_WT1]
  Control System 2/1(Grid_conv_pulses) -> [Grid_conv_pulses_WT2]
  Control System 2/2(Rotor_conv_pulses) -> [Rotor_conv_pulses_WT2]
  [Rotor_Iabc_WT3] -> Control System 3/4(Rotor_Iabc)
  [Grid_conv_Iabc_WT1] -> Control System 1/3(Grid_Iabc)
  Control System 4/3(Pitch) -> [Pitch_WT4]
  Control System 4/2(Rotor_conv_pulses) -> [Rotor_conv_pulses_WT4]
  [VDC_WT2] -> Control System 2/5(Vdc_V)
  [Rotor_Angle_WT1] -> Control System 1/7(angle_rotor_rad)
  [Q_ref_WT1] -> Control System 1/6(Qref1)
  [VDC_WT3] -> Control System 3/5(Vdc_V)
  Control System 3/3(Pitch) -> [Pitch_WT3]
  [Stator_Iabc_WT3] -> Control System 3/2(Stator_Iabc)
  [Rotor_wm_WT3] -> Control System 3/8(wr)
  [Rotor_Angle_WT3] -> Control System 3/7(angle_rotor_rad)
  [Stator_Iabc_WT1] -> Control System 1/2(Stator_Iabc)
  [Q_ref_WT3] -> Control System 3/6(Qref1)
  [Vabc_WT2] -> Control System 2/1(Vabc)
  [Vabc_WT3] -> Control System 3/1(Vabc)
  [Rotor_Iabc_WT1] -> Control System 1/4(Rotor_Iabc)
  [Rotor_Angle_WT2] -> Control System 2/7(angle_rotor_rad)
  [Stator_Iabc_WT2] -> Control System 2/2(Stator_Iabc)
  [Grid_conv_Iabc_WT2] -> Control System 2/3(Grid_Iabc)
  [VDC_WT4] -> Control System 4/5(Vdc_V)
  [Rotor_Iabc_WT2] -> Control System 2/4(Rotor_Iabc)
  [Vabc_WT4] -> Control System 4/1(Vabc)
  [Grid_conv_Iabc_WT4] -> Control System 4/3(Grid_Iabc)
  [Rotor_wm_WT2] -> Control System 2/8(wr)
  [Rotor_Iabc_WT4] -> Control System 4/4(Rotor_Iabc)
  Control System 1/2(Rotor_conv_pulses) -> [Rotor_conv_pulses_WT1]
  Control System 2/3(Pitch) -> [Pitch_WT2]
  [VDC_WT1] -> Control System 1/5(Vdc_V)
  Control System 3/1(Grid_conv_pulses) -> [Grid_conv_pulses_WT3]
  Control System 1/1(Grid_conv_pulses) -> [Grid_conv_pulses_WT1]
  Control System 3/2(Rotor_conv_pulses) -> [Rotor_conv_pulses_WT3]
  [Q_ref_WT4] -> Control System 4/6(Qref1)
  [Rotor_Angle_WT4] -> Control System 4/7(angle_rotor_rad)
  [Rotor_wm_WT4] -> Control System 4/8(wr)
  Control System 1/4(PQ) -> [PQ_WT1]
  Control System 2/4(PQ) -> [PQ_WT2]
  Control System 3/4(PQ) -> [PQ_WT3]
  Control System 4/4(PQ) -> [PQ_WT4]

== system 43_BusNetworkElectricityTransmissionModel/400 kV Solar Farm/DC//DC Boost Converter/MPPT ==
  PV_Current : Inport
  PV_Voltage : Inport  Port=2
  Add : Sum  Inputs=+-
  Deblock : Step  Time=0.5  SampleTime=0
  Duty Cycle : Constant  Value=Di
  "MPPT " : Subsystem
  PWM Generator (DC-DC) : spsPWMGeneratorDCDCLib/PWM Generator (DC-DC)  Fsw=fp  Ts=Tp
  Saturation : Saturate  UpperLimit=1  LowerLimit=0
  Pulses : Outport
  tag scope: D1=global
  wires:
  "MPPT "/1(delta D) -> Add/2
  Saturation/1 -> PWM Generator (DC-DC)/1, [D1]
  PV_Voltage/1 -> "MPPT "/2(PV_Voltage)
  Add/1 -> Saturation/1
  Deblock/1 -> "MPPT "/3(Switch port)
  Duty Cycle/1 -> Add/1
  PV_Current/1 -> "MPPT "/1(PV_Current)
  PWM Generator (DC-DC)/1 -> Pulses/1

== system 43_BusNetworkElectricityTransmissionModel/400 kV Solar Farm/DC//DC Boost Converter/Pmean Calculation ==
  Product1 : Product
  W to KW : Gain  Gain=1/1000
  tag scope: Pmean_PV1=global
  wires:
  Product1/1 -> W to KW/1
  [Imean_PV1] -> Product1/2
  [Vmean_PV1] -> Product1/1
  W to KW/1 -> [Pmean_PV1]

== system 43_BusNetworkElectricityTransmissionModel/400 kV Solar Farm/DC//DC Boost Converter1/MPPT ==
  PV_Current : Inport
  PV_Voltage : Inport  Port=2
  Add : Sum  Inputs=+-
  Deblock : Step  Time=0.5  SampleTime=0
  Duty Cycle : Constant  Value=Di
  "MPPT " : Subsystem
  PWM Generator (DC-DC) : spsPWMGeneratorDCDCLib/PWM Generator (DC-DC)  Fsw=fp  Ts=Tp
  Saturation : Saturate  UpperLimit=1  LowerLimit=0
  Pulses : Outport
  tag scope: D2=global
  wires:
  "MPPT "/1(delta D) -> Add/2
  Saturation/1 -> PWM Generator (DC-DC)/1, [D2]
  PV_Voltage/1 -> "MPPT "/2(PV_Voltage)
  Add/1 -> Saturation/1
  Deblock/1 -> "MPPT "/3(Switch port)
  Duty Cycle/1 -> Add/1
  PV_Current/1 -> "MPPT "/1(PV_Current)
  PWM Generator (DC-DC)/1 -> Pulses/1

== system 43_BusNetworkElectricityTransmissionModel/400 kV Solar Farm/DC//DC Boost Converter1/Pmean Calculation ==
  Product1 : Product
  W to KW : Gain  Gain=1/1000
  tag scope: Pmean_PV2=global
  wires:
  Product1/1 -> W to KW/1
  [Imean_PV2] -> Product1/2
  [Vmean_PV2] -> Product1/1
  W to KW/1 -> [Pmean_PV2]

== system 43_BusNetworkElectricityTransmissionModel/400 kV Solar Farm/DC//DC Boost Converter2/MPPT ==
  PV_Current : Inport
  PV_Voltage : Inport  Port=2
  Add : Sum  Inputs=+-
  Deblock : Step  Time=0.5  SampleTime=0
  Duty Cycle : Constant  Value=Di
  "MPPT " : Subsystem
  PWM Generator (DC-DC) : spsPWMGeneratorDCDCLib/PWM Generator (DC-DC)  Fsw=fp  Ts=Tp
  Saturation : Saturate  UpperLimit=1  LowerLimit=0
  Pulses : Outport
  tag scope: D3=global
  wires:
  "MPPT "/1(delta D) -> Add/2
  Saturation/1 -> PWM Generator (DC-DC)/1, [D3]
  PV_Voltage/1 -> "MPPT "/2(PV_Voltage)
  Add/1 -> Saturation/1
  Deblock/1 -> "MPPT "/3(Switch port)
  Duty Cycle/1 -> Add/1
  PV_Current/1 -> "MPPT "/1(PV_Current)
  PWM Generator (DC-DC)/1 -> Pulses/1

== system 43_BusNetworkElectricityTransmissionModel/400 kV Solar Farm/DC//DC Boost Converter2/Pmean Calculation ==
  Product1 : Product
  W to KW : Gain  Gain=1/1000
  tag scope: Pmean_PV3=global
  wires:
  Product1/1 -> W to KW/1
  [Imean_PV3] -> Product1/2
  [Vmean_PV3] -> Product1/1
  W to KW/1 -> [Pmean_PV3]

== system 43_BusNetworkElectricityTransmissionModel/400 kV Solar Farm/DC//DC Boost Converter3/MPPT ==
  PV_Current : Inport
  PV_Voltage : Inport  Port=2
  Add : Sum  Inputs=+-
  Deblock : Step  Time=0.5  SampleTime=0
  Duty Cycle : Constant  Value=Di
  "MPPT " : Subsystem
  PWM Generator (DC-DC) : spsPWMGeneratorDCDCLib/PWM Generator (DC-DC)  Fsw=fp  Ts=Tp
  Saturation : Saturate  UpperLimit=1  LowerLimit=0
  Pulses : Outport
  tag scope: D4=global
  wires:
  "MPPT "/1(delta D) -> Add/2
  Saturation/1 -> PWM Generator (DC-DC)/1, [D4]
  PV_Voltage/1 -> "MPPT "/2(PV_Voltage)
  Add/1 -> Saturation/1
  Deblock/1 -> "MPPT "/3(Switch port)
  Duty Cycle/1 -> Add/1
  PV_Current/1 -> "MPPT "/1(PV_Current)
  PWM Generator (DC-DC)/1 -> Pulses/1

== system 43_BusNetworkElectricityTransmissionModel/400 kV Solar Farm/DC//DC Boost Converter3/Pmean Calculation ==
  Product1 : Product
  W to KW : Gain  Gain=1/1000
  tag scope: Pmean_PV4=global
  wires:
  Product1/1 -> W to KW/1
  [Imean_PV4] -> Product1/2
  [Vmean_PV4] -> Product1/1
  W to KW/1 -> [Pmean_PV4]

== system 43_BusNetworkElectricityTransmissionModel/400 kV Solar Farm/VSC Control/Current Regulator ==
  VdVq_mes : Inport  PortDimensions=2
  IdIq_mes : Inport  Port=2  PortDimensions=2
  IdIq_ref : Inport  Port=3  PortDimensions=2
  Add1 : Sum  Inputs=++-
  Add2 : Sum
  Add3 : Sum  Inputs=+++
  Demux : Demux  Outputs=2
  Demux1 : Demux  Outputs=2
  Ltot_pu1 : Gain  Gain=Ltot_pu  SaturateOnIntegerOverflow=on  OutDataTypeStr=Inherit: Same as input  ParamDataTypeStr=Inherit: Same as input
  Ltot_pu2 : Gain  Gain=Ltot_pu  SaturateOnIntegerOverflow=on  OutDataTypeStr=Inherit: Same as input  ParamDataTypeStr=Inherit: Same as input
  Mux : Mux  Inputs=2
  PI : slpidlib/PID Controller  Controller=PI  Form=Parallel  TimeDomain=Discrete-time  UseExternalTs=off  SampleTime=Ts  IntegratorMethod=Forward Euler  FilterMethod=Forward Euler  ControllerParametersSource=internal  P=Kp_Ireg  I=Ki_Ireg  UseKiTs=off  D=0  N=100  UseFilter=on  TunerSelectOption=Transfer Function Based (PID Tuner App)  InitialConditionSource=internal  InitialConditionForIntegrator=0  InitialConditionForFilter=0  DifferentiatorICPrevScaledInput=0  ExternalReset=none  TrackingMode=off  Kt=1  LimitOutput=on  SatLimitsSource=internal  UpperSaturationLimit=2  LowerSaturationLimit=-2  LinearizeAsGain=off  AntiWindupMode=none  Kb=1  LimitIntegrator=off  UpperIntegratorSaturationLimit=inf  LowerIntegratorSaturationLimit=-inf  POutMin=[]  POutMax=[]  IOutMin=[]  IOutMax=[]  DOutMin=[]  DOutMax=[]  NOutMin=[]  NOutMax=[]  SumOutMin=[]  SumOutMax=[]  SaturationOutMin=[]  SaturationOutMax=[]  PParamMin=[]  PParamMax=[]  IParamMin=[]  IParamMax=[]  DParamMin=[]  DParamMax=[]  NParamMin=[]  NParamMax=[]  KbParamMin=[]  KbParamMax=[]  KtParamMin=[]  KtParamMax=[]  KbOutMin=[]  KbOutMax=[]  KtOutMin=[]  KtOutMax=[]  IntegratorOutMin=[]  IntegratorOutMax=[]  FilterOutMin=[]  FilterOutMax=[]  SumI1OutMin=[]  SumI1OutMax=[]  SumI2OutMin=[]  SumI2OutMax=[]  SumI3OutMin=[]  SumI3OutMax=[]  SumI4OutMin=[]  SumI4OutMax=[]  SumDOutMin=[]  SumDOutMax=[]  DifferentiatorOutMin=[]  DifferentiatorOutMax=[]  FilterDiffOutCoefMin=[]  FilterDiffOutCoefMax=[]  ReciprocalOutMin=[]  ReciprocalOutMax=[]  SumDenOutMin=[]  SumDenOutMax=[]  SumNumOutMin=[]  SumNumOutMax=[]  DivideOutMin=[]  DivideOutMax=[]  UdiffTsProdOutMin=[]  UdiffTsProdOutMax=[]  NTsProdOutMin=[]  NTsProdOutMax=[]  UintegralTsProdOutMin=[]  UintegralTsProdOutMax=[]  UngainTsProdOutMin=[]  UngainTsProdOutMax=[]  ClampingZeroOutDataTypeStr=Inherit: Inherit via back propagation  ClampingZeroOutMin=[]  ClampingZeroOutMax=[]  FilterDenConstantOutDataTypeStr=Inherit: Inherit via back propagation  FilterDenConstantOutMin=[]  FilterDenConstantOutMax=[]  PCopyOutDataTypeStr=Inherit: Inherit via back propagation  PCopyOutMin=[]  PCopyOutMax=[]  NCopyOutDataTypeStr=Inherit: Inherit via back propagation  NCopyOutMin=[]  NCopyOutMax=[]  IntegratorContinuousStateAttributes=''  IntegratorStateMustResolveToSignalObject=off  IntegratorRTWStateStorageClass=Auto  FilterContinuousStateAttributes=''  FilterStateMustResolveToSignalObject=off  FilterRTWStateStorageClass=Auto  ParallelPVariant=InternalParameters  IdealPVariant=Disabled  IVariant=InternalParameters  DVariant=Disabled  IntegratorVariant=Discrete  SatVariant=Enabled  AWVariant=Passthrough  PCopyVariant=Disabled  TRVariant=Disabled  FdbkBlocksVariant=Forward  IdealPFdbkVariant=Disabled  SatFdbkVariant=Disabled  DerivativeFilterVariant=Disabled  NVariant=Disabled  NCopyVariant=Disabled_SignalSpec  FilterICVariant=Disabled  IntegratorICVariant=InternalICs  ExternalResetVariant=Disabled  TRSumVariant=Passthrough  SumFdbkVariant=Disabled  SumVariant=Sum_PI  TsampFilterVariant=InternalTs  TsampNgainVariant=Passthrough  TsampIntegralVariant=Disabled_SignalSpec  ExternalSaturationOutDataTypeStr=Inherit: Same as second input
  PI_Ireg1 : Scope
  Rtot_pu1 : Gain  Gain=Rtot_pu  SaturateOnIntegerOverflow=on  OutDataTypeStr=Inherit: Same as input  ParamDataTypeStr=Inherit: Same as input
  Rtot_pu5 : Gain  Gain=Rtot_pu  SaturateOnIntegerOverflow=on  OutDataTypeStr=Inherit: Same as input  ParamDataTypeStr=Inherit: Same as input
  Saturation : Saturate  UpperLimit=2  LowerLimit=-2
  Sum : Sum  Inputs=|-+
  VdVq_conv : Outport  VectorParamsAs1DForOutWhenUnconnected=off
  wires:
  Mux/1 -> PI_Ireg1/1, Add2/2
  PI/1 -> Add2/1  "PI"
  Sum/1 -> PI/1
  IdIq_ref/1 -> Sum/2, Demux1/1
  IdIq_mes/1 -> Sum/1
  Add2/1 -> Saturation/1
  Saturation/1 -> VdVq_conv/1
  VdVq_mes/1 -> Demux/1
  Demux/1 -> Add1/1
  Rtot_pu1/1 -> Add1/2
  Demux1/1 -> Rtot_pu1/1, Ltot_pu2/1
  Ltot_pu1/1 -> Add1/3
  Demux1/2 -> Ltot_pu1/1, Rtot_pu5/1
  Rtot_pu5/1 -> Add3/2
  Ltot_pu2/1 -> Add3/3
  Add1/1 -> Mux/1  "Feedforward"
  Demux/2 -> Add3/1
  Add3/1 -> Mux/2

== system 43_BusNetworkElectricityTransmissionModel/400 kV Solar Farm/VSC Control/PLL & Measurements ==
  Vabc_prim : Inport
  Iabc_prim : Inport  Port=2
  PLL (3ph) : spsPLL3phLib/PLL (3ph)  Fmin=45  Par_Init="[-0.57  Fnom]"  ParK=[180, 3200, 1]  TcD=Ts  MaxRateChangeFreq=12  FilterCutOffFreq=25  Ts=Ts  AGC=on
  Selector1 : Selector  InputPortWidth=3  IndexOptions=Index vector (dialog)  Indices=[1 2]  OutputSizes=1
  Selector2 : Selector  InputPortWidth=3  IndexOptions=Index vector (dialog)  Indices=[1 2]  OutputSizes=1
  Terminator : Terminator
  V->pu : Gain  Gain=1/(Vnom_prim*sqrt(2)/sqrt(3))  SaturateOnIntegerOverflow=on  OutDataTypeStr=Inherit: Same as input  ParamDataTypeStr=Inherit: Same as input
  V->pu1 : Gain  Gain=Vnom_prim*sqrt(3)/Pnom/sqrt(2)  SaturateOnIntegerOverflow=on  OutDataTypeStr=Inherit: Same as input  ParamDataTypeStr=Inherit: Same as input
  abc to dq0 : spsabctodq0Lib/abc to dq0  Alignment=90 degrees behind phase A axis
  abc to dq1 : spsabctodq0Lib/abc to dq0  Alignment=90 degrees behind phase A axis
  wt : Outport  VectorParamsAs1DForOutWhenUnconnected=off
  VdVq_prim : Outport  Port=2  VectorParamsAs1DForOutWhenUnconnected=off
  IdIq_prim : Outport  Port=3  VectorParamsAs1DForOutWhenUnconnected=off
  wires:
  V->pu1/1 -> abc to dq1/1
  V->pu/1 -> PLL (3ph)/1, abc to dq0/1
  abc to dq1/1 -> Selector1/1
  Vabc_prim/1 -> V->pu/1
  Iabc_prim/1 -> V->pu1/1
  abc to dq0/1 -> Selector2/1
  Selector2/1 -> VdVq_prim/1
  Selector1/1 -> IdIq_prim/1
  PLL (3ph)/2 -> wt/1, abc to dq1/2, abc to dq0/2
  PLL (3ph)/1 -> Terminator/1
